simulink model "BESSmodel_EMT"  (R2019a)
settings: Solver=FixedStepAuto  SolverName=VariableStepAuto  StartTime=0.0  StopTime=10  RelTol=1e-3
undefined symbols (not defined in the file): D11, Delta, Ion, Lithium
libraries: powerlib x24, powerlib_meascontrol x15, simulink x9, eeGeneralControl x8, electricdrivelib x1
(part 1 of 2)
settings Model: Creator=rodne  LastModifiedBy=iq22022
settings DebuggingCC: UnderspecifiedInitializationDetection=Classic  MergeDetectMultiDrivingBlocksExec=none  UnconnectedInputMsg=none  UnconnectedOutputMsg=none  UnconnectedLineMsg=none  SFMachineParentedDataDiag=error
settings ModelReferenceCC: PropagateSignalLabelsOutOfModel=off

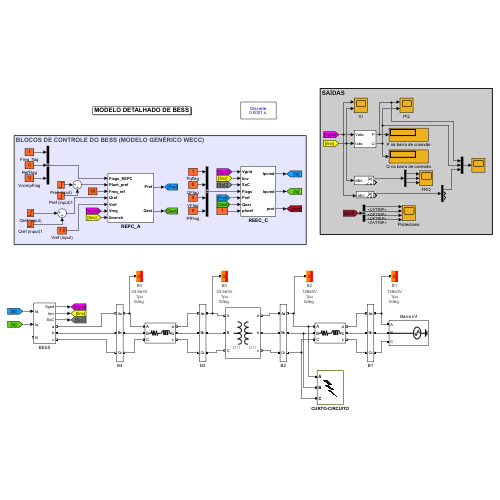
[thumbnail: Simulink's stored preview of the top-level diagram]
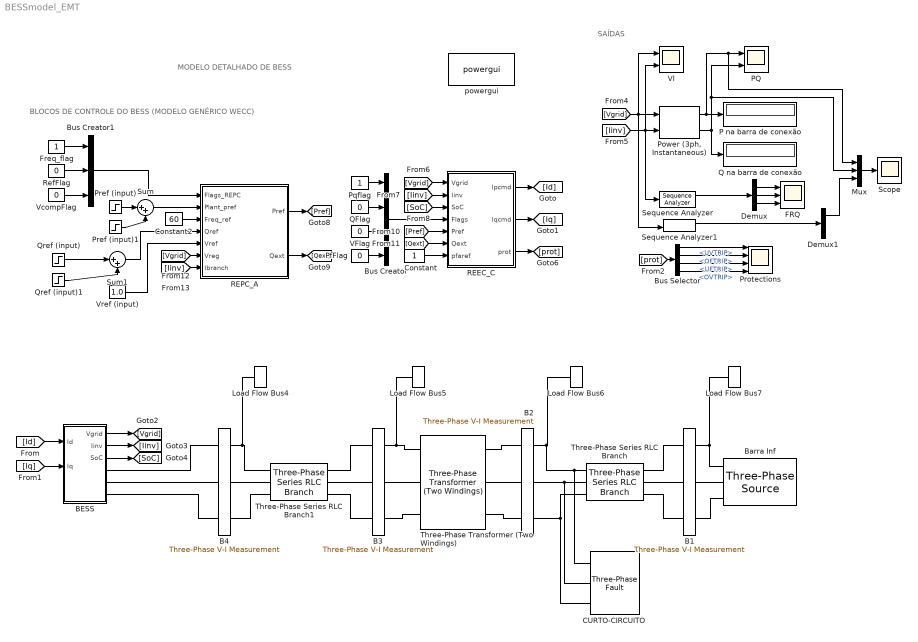
== system BESSmodel_EMT ==
  note: MODELO DETALHADO DE BESS
  note: SAÍDAS
  note: BLOCOS DE CONTROLE DO BESS (MODELO GENÉRICO WECC)
  B{1..4} (4 alike) : powerlib/Measurements/Three-Phase V-I Measurement  VoltageMeasurement=no  SetLabelV=off  LabelV=Vabc  Vpu=off  VpuLL=off  CurrentMeasurement=no  SetLabelI=off  LabelI=Iabc  Ipu=off  Pbase=100e6  Vbase=500e3  OutputType=Complex  PhasorSimulation=off  PSBequivalent=0
  BESS : Subsystem
  Barra Inf : powerlib/Electrical Sources/Three-Phase Source  InternalConnection=Yg  VoltagePhases=off  Voltage=138e3  PhaseAngle=0  Voltage_phases=[25e3 25e3 25e3]/sqrt(3)  PhaseAngles_phases=[0 -120 +120]  Frequency=60  NonIdealSource=off  SpecifyImpedance=off  Resistance=0.8929  Inductance=16.58e-3  ShortCircuitLevel=100e6  BaseVoltage=138e3  XRratio=7  BusType=swing  Pref=10e3  Qref=0  Prefabc=[10e3, 10e3, 10e3]  Qrefabc=[0, 0, 0]  Qmin=-inf  Qmax=inf
  Bus Creator : BusCreator  Inputs=4
  Bus Creator1 : BusCreator  Inputs=3
  Bus Selector : BusSelector  OutputSignals=UVTRIP,OFTRIP,UFTRIP,OVTRIP
  CURTO-CIRCUITO : powerlib/Elements/Three-Phase Fault  InitialStates=0  FaultA=on  FaultB=off  FaultC=off  GroundFault=on  SwitchTimes="[5.0  6.0]"  External=off  SwitchStatus=NaN  FaultResistance=60  GroundResistance=0.01  SnubberResistance=1e6  SnubberCapacitance=inf  Measurements=None
  Constant : Constant
  Constant2 : Constant  Value=60
  Demux : Demux  Outputs=3
  Demux1 : Demux  Outputs=3
  FRQ : Scope  NumInputPorts=3
  Freq_flag : Constant
  Load Flow Bus4 : powerlib/Measurements/Load Flow Bus  LConnTagsString=a  Phases=single  Connectors=on one side  ID=B4  Vbase=34.5e3  Vref=0.97  Vangle=0  VLF=1  VLFb=1  VLFc=1  angleLF=0  angleLFb=0  angleLFc=0
  Load Flow Bus5 : powerlib/Measurements/Load Flow Bus  LConnTagsString=a  Phases=single  Connectors=on one side  ID=B3  Vbase=34.5e3  Vref=1  Vangle=0  VLF=1  VLFb=1  VLFc=1  angleLF=0  angleLFb=0  angleLFc=0
  Load Flow Bus6 : powerlib/Measurements/Load Flow Bus  LConnTagsString=a  Phases=single  Connectors=on one side  ID=B2  Vbase=138e3  Vref=1  Vangle=0  VLF=1  VLFb=1  VLFc=1  angleLF=0  angleLFb=0  angleLFc=0
  Load Flow Bus7 : powerlib/Measurements/Load Flow Bus  LConnTagsString=a  Phases=single  Connectors=on one side  ID=B1  Vbase=138e3  Vref=1  Vangle=0  VLF=1  VLFb=1  VLFc=1  angleLF=0  angleLFb=0  angleLFc=0
  Mux : Mux  Inputs=3
  P na barra de conexão : Display
  PQ : Scope  NumInputPorts=2
  PfFlag : Constant  Value=0
  "Power (3ph, Instantaneous)" : powerlib_meascontrol/Measurements/Power (3ph, Instantaneous)
  Pqflag : Constant
  Pref (input) : Step  After=1.0  SampleTime=0
  Pref (input)1 : Step  Time=10  After=0  SampleTime=0
  Protections : Scope  NumInputPorts=4
  Q na barra de conexão : Display
  QFlag : Constant  Value=0
  Qref (input) : Step  Time=15  After=0  SampleTime=0
  Qref (input)1 : Step  Time=25  After=0  SampleTime=0
  REEC_C : Subsystem
  REPC_A : Subsystem
  RefFlag : Constant  Value=0
  Scope : Scope
  Sequence Analyzer : powerlib_meascontrol/Measurements/Sequence Analyzer  Freq=60  n=1  seq=Positive Negative Zero  InInit=[1, 0]  Ts=0
      settings: SourceProductBaseCode=PS
  Sequence Analyzer1 : powerlib_meascontrol/Measurements/Sequence Analyzer  Freq=60  n=1  seq=Positive Negative Zero  InInit=[1, 0]  Ts=0
      settings: SourceProductBaseCode=PS
  Sum : Sum  Inputs=|++
  Sum1 : Sum  Inputs=|++
  Three-Phase Series RLC Branch : powerlib/Elements/Three-Phase Series RLC Branch  LConnTagsString=A|B|C  RConnTagsString=A|B|C  BranchType=RL  Resistance=28.1667  Inductance=281.6667/(2*pi*60)  Capacitance=1e-6  Measurements=None
  Three-Phase Series RLC Branch1 : powerlib/Elements/Three-Phase Series RLC Branch  LConnTagsString=A|B|C  RConnTagsString=A|B|C  BranchType=RL  Resistance=0.0119  Inductance=0.1190/(2*pi*60)  Capacitance=1e-6  Measurements=None
  Three-Phase Transformer (Two Windings) : powerlib/Elements/Three-Phase Transformer (Two Windings)  Winding1Connection=Delta (D11)  Winding2Connection=Delta (D11)  CoreType=Three single-phase transformers  SetSaturation=off  Hysteresis=off  DataFile='hysteresis'  SetInitialFlux=off  Measurements=None  UNITS=pu  NominalPower=[ 6e6 , 60 ]  Winding1=[34.5e+03 0.0001/2 0.06/(2*pi*60)/2]  Winding2=[138e+03 0.0001/2 0.06/(2*pi*60)/2]  Rm=499.98  Lm=500  L0=0.5  Saturation=[0 0;0.0024 1.2;1 1.52]  InitialFluxes=[ 0.8 , -0.8 , 0.7 ]  BreakLoop=off  DiscreteSolver=Trapezoidal iterative  DataType=off  TransfoNumber=1
  VFlag : Constant  Value=0
  VI : Scope  NumInputPorts=2
  VcompFlag : Constant  Value=0
  Vref (input) : Constant  Value=1.0
  powergui : powerlib/powergui  Priority=1  SimulationMode=Discrete  SampleTime=100e-6  frequency=60  Iterations=50  frequencyindice=60  Pbase=100e6  ErrMax=1e-4  UnitsV=kV  UnitsW=MW  buscounter=0  FunctionMessages=off  echomessages=off  EnableUseOfTLC=off  CurrentSourceSwitches=off  DisableSnubberDevices=off  DisableRonSwitches=off  DisableVfSwitches=off  DisplayEquations=off  AutomaticDiscreteSolvers=off  SolverType=Tustin/Backward Euler (TBE)  Interpol=off  ExternalGateDelay=off  methode=off  Ts=100  x0status=blocks  SPID=on  SwTol=0  HookPort=off  NonlinearTolerance=1e-4  nMaxIteration=100  ContinueOnMaxIteration=off  RestoreLinks=warning  ResistiveCurrentMeasurement=off  Frange=[0:2:500]  Ylog=off  Xlog=on  ShowGrid=off  save=off  variable=ZData  structure=0  ZoomFFT=off  StartTime=0.0  cycles=1  DisplayStyle=1  fundamental=60  FreqAxis=off  MaxFrequency=1000  frequencyindicesteady=1  RmsSteady=1  display=off
  wires:
  "Power (3ph, Instantaneous)"/1 -> Mux/1, PQ/1, P na barra de conexão/1
  "Power (3ph, Instantaneous)"/2 -> PQ/2, Mux/2, Q na barra de conexão/1
  REEC_C/1(Ipcmd) -> [Id]
  REEC_C/2(Iqcmd) -> [Iq]
  [Vgrid] -> Sequence Analyzer1/1, VI/1, "Power (3ph, Instantaneous)"/1
  [Iinv] -> Sequence Analyzer/1, VI/2, "Power (3ph, Instantaneous)"/2
  [Vgrid] -> REEC_C/1(Vgrid)
  [Iinv] -> REEC_C/2(Iinv)
  [SoC] -> REEC_C/3(SoC)
  Pqflag/1 -> Bus Creator/1
  QFlag/1 -> Bus Creator/2
  PfFlag/1 -> Bus Creator/4
  VFlag/1 -> Bus Creator/3
  Bus Creator/1 -> REEC_C/4(Flags)
  Constant/1 -> REEC_C/7(pfaref)
  [Id] -> BESS/1(Id)
  [Iq] -> BESS/2(Iq)
  BESS/1(Vgrid) -> [Vgrid]
  BESS/2(Iinv) -> [Iinv]
  BESS/3(SoC) -> [SoC]
  Freq_flag/1 -> Bus Creator1/1
  RefFlag/1 -> Bus Creator1/2
  VcompFlag/1 -> Bus Creator1/3
  Bus Creator1/1 -> REPC_A/1(Flags_REPC)
  REPC_A/1(Pref) -> [Pref]
  REPC_A/2(Qext) -> [Qext]
  Constant2/1 -> REPC_A/3(Freq_ref)
  Vref (input)/1 -> REPC_A/5(Vref)
  [Pref] -> REEC_C/5(Pref)
  [Vgrid] -> REPC_A/6(Vreg)
  [Iinv] -> REPC_A/7(Ibranch)
  [Qext] -> REEC_C/6(Qext)
  REEC_C/3(prot) -> [prot]
  [prot] -> Bus Selector/1
  Bus Selector/1 -> Protections/1  "<UVTRIP>"
  Bus Selector/2 -> Protections/2  "<OFTRIP>"
  Bus Selector/3 -> Protections/3  "<UFTRIP>"
  Bus Selector/4 -> Protections/4  "<OVTRIP>"
  Sequence Analyzer/1 -> Demux/1
  Demux/1 -> FRQ/1
  Demux/2 -> FRQ/2
  Demux/3 -> FRQ/3
  Sum/1 -> REPC_A/2(Plant_pref)
  Pref (input)/1 -> Sum/1
  Pref (input)1/1 -> Sum/2
  Sum1/1 -> REPC_A/4(Qref)
  Qref (input)/1 -> Sum1/1
  Qref (input)1/1 -> Sum1/2
  Sequence Analyzer1/1 -> Demux1/1
  Mux/1 -> Scope/1
  Demux1/1 -> Mux/3
  connections:
  BESS/RConn1 -- B4/LConn1
  B4/LConn2 -- BESS/RConn2
  BESS/RConn3 -- B4/LConn3
  B3/RConn1 -- Load Flow Bus5/LConn1 -- Three-Phase Transformer (Two Windings)/LConn1
  Load Flow Bus7/LConn1 -- Barra Inf/RConn1 -- B1/RConn1
  B2/RConn1 -- CURTO-CIRCUITO/LConn1 -- Three-Phase Series RLC Branch/LConn1 -- Load Flow Bus6/LConn1
  B4/RConn1 -- Three-Phase Series RLC Branch1/LConn1 -- Load Flow Bus4/LConn1
  Three-Phase Series RLC Branch1/LConn2 -- B4/RConn2
  B3/RConn3 -- Three-Phase Transformer (Two Windings)/LConn3
  B3/RConn2 -- Three-Phase Transformer (Two Windings)/LConn2
  Three-Phase Series RLC Branch/RConn2 -- B1/LConn2
  Three-Phase Series RLC Branch1/RConn3 -- B3/LConn3
  B2/LConn3 -- Three-Phase Transformer (Two Windings)/RConn3
  B2/LConn1 -- Three-Phase Transformer (Two Windings)/RConn1
  Three-Phase Series RLC Branch/LConn2 -- CURTO-CIRCUITO/LConn2 -- B2/RConn2
  Three-Phase Series RLC Branch/RConn3 -- B1/LConn3
  Three-Phase Series RLC Branch1/RConn2 -- B3/LConn2
  Three-Phase Series RLC Branch1/RConn1 -- B3/LConn1
  Three-Phase Series RLC Branch/RConn1 -- B1/LConn1
  B2/LConn2 -- Three-Phase Transformer (Two Windings)/RConn2
  Three-Phase Series RLC Branch/LConn3 -- CURTO-CIRCUITO/LConn3 -- B2/RConn3
  Three-Phase Series RLC Branch1/LConn3 -- B4/RConn3
  Barra Inf/RConn2 -- B1/RConn2
  Barra Inf/RConn3 -- B1/RConn3

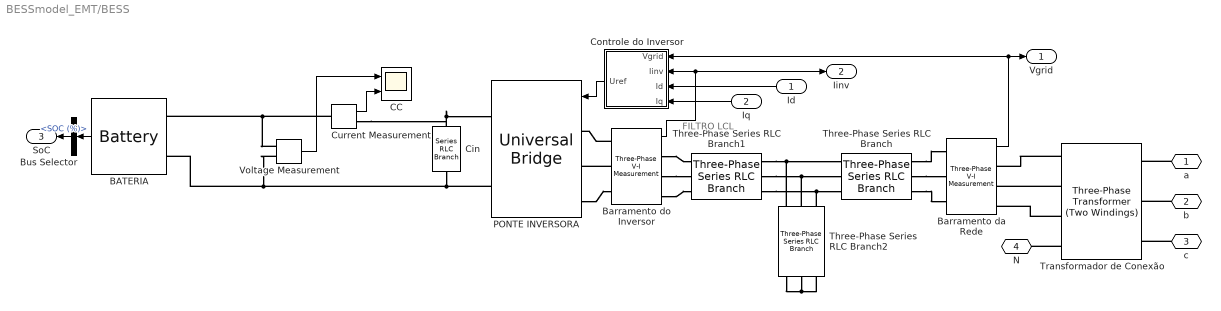
== system BESSmodel_EMT/BESS ==
  note: FILTRO LCL
  Id : Inport
  Iq : Inport  Port=2
  BATERIA : electricdrivelib/Extra Sources/Battery  BatType=Lithium-Ion  ShowTempParam=off  ThermalPreset=no  ShowAgeParam=off  NomV=1332  NomQ=280  SOC=70  Batt_Tr=30  PresetModel=off  MaxQ=280  MinV=999  FullV=1550.4309  Dis_rate=121.7391  R=0.047571*2.0  Normal_OP=253.2174  expZone="[1439.074      13.756522]"  current=[6.5 13 32.5]  Units=Time  Tci=20  NomT=20  T2=-30  MaxQ2=4.8  FullV2=7.1  Normal_OP2=5.655  expZone2="[6.58           1]"  Rca=0.6  ti=2000  Dp=0  Neq0=0  Tsim=1e6  Ta1=25  Qeol=5.4*0.9  Reol=0.013333*1.2  Char_age=[2.3478, 3]  Dis_age=[2.3478, 10]  N1=1500  N2=10500  N3=1000  N4=1400  Ta2=45  N5=950
  Barramento da Rede : powerlib/Measurements/Three-Phase V-I Measurement  VoltageMeasurement=phase-to-phase  SetLabelV=off  LabelV=Vabc  Vpu=off  VpuLL=on  CurrentMeasurement=no  SetLabelI=off  LabelI=Iabc  Ipu=off  Pbase=100e6  Vbase=690  OutputType=Complex  PhasorSimulation=off  PSBequivalent=0
  Barramento do Inversor : powerlib/Measurements/Three-Phase V-I Measurement  VoltageMeasurement=no  SetLabelV=off  LabelV=Vabc  Vpu=off  VpuLL=off  CurrentMeasurement=yes  SetLabelI=off  LabelI=Iabc  Ipu=on  Pbase=100e6  Vbase=690e3  OutputType=Complex  PhasorSimulation=off  PSBequivalent=0
  Bus Selector : BusSelector  OutputSignals=SOC (%)
  CC : Scope  NumInputPorts=2
  Cin : powerlib/Elements/Series RLC Branch  LConnTagsString=__new0  RConnTagsString=__new0  BranchType=RC  Resistance=0.0025  Inductance=1e-3  SetiL0=off  InitialCurrent=0  Capacitance=100e-6  Setx0=off  InitialVoltage=0  Measurements=None
  Controle do Inversor : Subsystem  mask(Direct-Quadrature Synchronous Reference Frame Controller){VDC=1332, f=60, fsw=10000, L=1000e-6, kp=5, ki=5000}
      mask prompts: VDC "DC Link Voltage (V)"; f "Grid Frequency (Hz)"; fsw "Switching Frequency (Hz)"; L "Filter Inductance (H)"; kp "Proportional Gain"; ki "Integral Gain"
      mask help:
      | Developed by Rodney Tan (PhD)
      | Version 1.0 (Nov 2021)
      |
      | This model demonstrate the operation of 3 phase grid connected inverter using Direct-Quadrature Synchronous Reference Frame Control.
      |
      | SPWM is use to switch the IGBT inverter bridge.
      |
      | The controller allows user to set the DC link voltage, active and reactive current for the inverter to be injected to the grid.
      |
      | The scope monitor the grid inverter output voltage and current waveform.
      |
      | The display monitor the active and reactive power injected to the grid.
      mask DialogControl Container3 Prompt: PI Controller Setting
  Current Measurement : powerlib/Measurements/Current Measurement  PhasorSimulation=off  OutputType=Complex  PSBequivalent=0
  PONTE INVERSORA : powerlib/Power Electronics/Universal Bridge  Arms=3  SnubberResistance=1e5  SnubberCapacitance=inf  Device=Average-model based VSC  Ron=1e-3  Lon=0  ForwardVoltages="[  0  0  ]"  ForwardVoltage=0  GTOparameters=[ 10e-6 , 20e-6 ]  IGBTparameters=[ 1e-6 , 2e-6 ]  Measurements=None  Measurements_2=None  converterType=Rectifier
  Three-Phase Series RLC Branch : powerlib/Elements/Three-Phase Series RLC Branch  LConnTagsString=A|B|C  RConnTagsString=A|B|C  BranchType=L  Resistance=1  Inductance=500e-6  Capacitance=1e-6  Measurements=None
  Three-Phase Series RLC Branch1 : powerlib/Elements/Three-Phase Series RLC Branch  LConnTagsString=A|B|C  RConnTagsString=A|B|C  BranchType=L  Resistance=1  Inductance=500e-6  Capacitance=1e-6  Measurements=None
  Three-Phase Series RLC Branch2 : powerlib/Elements/Three-Phase Series RLC Branch  LConnTagsString=A|B|C  RConnTagsString=A|B|C  BranchType=C  Resistance=1  Inductance=1e-3  Capacitance=700e-6  Measurements=None
  Transformador de Conexão : powerlib/Elements/Three-Phase Transformer (Two Windings)  Winding1Connection=Yn  Winding2Connection=Delta (D11)  CoreType=Three single-phase transformers  SetSaturation=off  Hysteresis=off  DataFile='hysteresis'  SetInitialFlux=off  Measurements=None  UNITS=pu  NominalPower=[ 34.5e6 , 60 ]  Winding1=[ 690 , 0.002 , 0.08 ]  Winding2=[ 34.5e3 , 0.002 , 0.08 ]  Rm=500  Lm=500  L0=0.5  Saturation=[ 0,0 ; 0.0024,1.2 ; 1.0,1.52 ]  InitialFluxes=[ 0.8 , -0.8 , 0.7 ]  BreakLoop=off  DiscreteSolver=Trapezoidal iterative  DataType=off  TransfoNumber=1
  Voltage Measurement : powerlib/Measurements/Voltage Measurement  PhasorSimulation=off  OutputType=Complex  PSBequivalent=0
  a : PMIOPort  Side=Right
  b : PMIOPort  Port=2  Side=Right
  c : PMIOPort  Port=3  Side=Right
  N : PMIOPort  Port=4  Side=Left
  Vgrid : Outport
  Iinv : Outport  Port=2
  SoC : Outport  Port=3
  wires:
  Id/1 -> Controle do Inversor/3(Id)
  Bus Selector/1 -> SoC/1  "<SOC (%)>"
  Iq/1 -> Controle do Inversor/4(Iq)
  Barramento da Rede/1 -> Vgrid/1, Controle do Inversor/1(Vgrid)
  Controle do Inversor/1(Uref) -> PONTE INVERSORA/1
  BATERIA/1 -> Bus Selector/1
  Barramento do Inversor/1 -> Controle do Inversor/2(Iinv), Iinv/1
  Voltage Measurement/1 -> CC/1
  Current Measurement/1 -> CC/2
  connections:
  Three-Phase Series RLC Branch1/RConn3 -- Three-Phase Series RLC Branch/LConn3 -- Three-Phase Series RLC Branch2/LConn3
  Transformador de Conexão/LConn2 -- Barramento da Rede/RConn2
  Three-Phase Series RLC Branch1/RConn2 -- Three-Phase Series RLC Branch/LConn2 -- Three-Phase Series RLC Branch2/LConn2
  PONTE INVERSORA/LConn3 -- Barramento do Inversor/LConn3
  b/RConn1 -- Transformador de Conexão/RConn2
  PONTE INVERSORA/RConn2 -- Voltage Measurement/LConn2 -- BATERIA/LConn2 -- Cin/RConn1
  Three-Phase Series RLC Branch2/RConn1 -- Three-Phase Series RLC Branch2/RConn2 -- Three-Phase Series RLC Branch2/RConn3
  Transformador de Conexão/LConn1 -- Barramento da Rede/RConn1
  Cin/LConn1 -- Current Measurement/RConn1 -- PONTE INVERSORA/RConn1
  Three-Phase Series RLC Branch1/RConn1 -- Three-Phase Series RLC Branch/LConn1 -- Three-Phase Series RLC Branch2/LConn1
  Transformador de Conexão/LConn4 -- N/RConn1
  c/RConn1 -- Transformador de Conexão/RConn3
  Barramento do Inversor/LConn2 -- PONTE INVERSORA/LConn2
  Barramento do Inversor/RConn1 -- Three-Phase Series RLC Branch1/LConn1
  Barramento do Inversor/RConn3 -- Three-Phase Series RLC Branch1/LConn3
  Barramento do Inversor/RConn2 -- Three-Phase Series RLC Branch1/LConn2
  Three-Phase Series RLC Branch/RConn2 -- Barramento da Rede/LConn2
  a/RConn1 -- Transformador de Conexão/RConn1
  Barramento do Inversor/LConn1 -- PONTE INVERSORA/LConn1
  Three-Phase Series RLC Branch/RConn1 -- Barramento da Rede/LConn1
  Transformador de Conexão/LConn3 -- Barramento da Rede/RConn3
  Three-Phase Series RLC Branch/RConn3 -- Barramento da Rede/LConn3
  Current Measurement/LConn1 -- Voltage Measurement/LConn1 -- BATERIA/LConn1

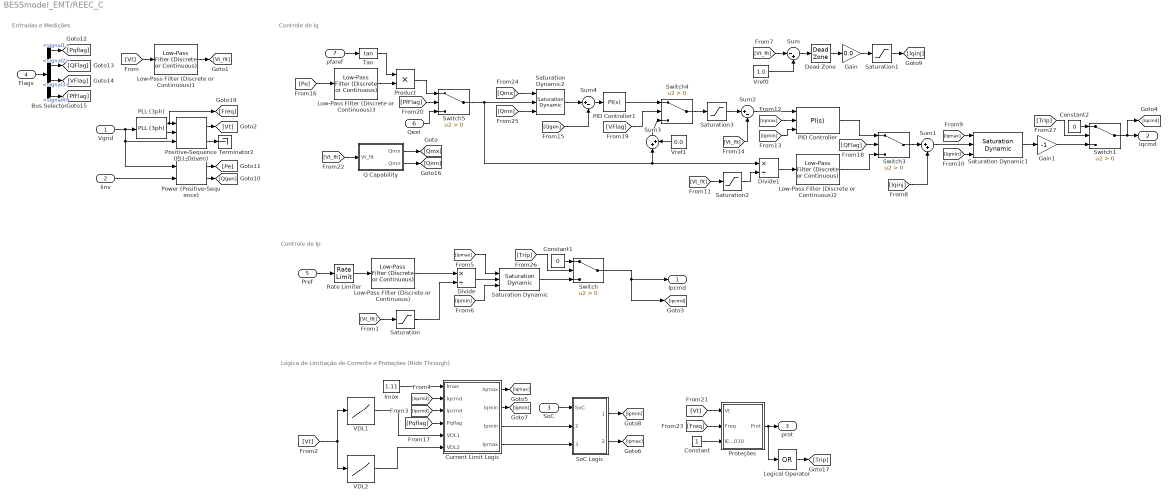
== system BESSmodel_EMT/REEC_C ==
  note: Entradas e Medições
  note: Controle de Iq
  note: Lógica de Limitação de Corrente e Proteções (Ride Through)
  note: Controle de Ip
  Vgrid : Inport
  Iinv : Inport  Port=2
  SoC : Inport  Port=3
  Flags : Inport  Port=4
  Pref : Inport  Port=5
  Qext : Inport  Port=6
  pfaref : Inport  Port=7
  Bus Selector : BusSelector  OutputSignals=signal1,signal2,signal3,signal4
  Constant : Constant
  Constant1 : Constant  Value=0
  Constant2 : Constant  Value=0
  Current Limit Logic : Subsystem
  Dead Zone : DeadZone  LowerValue=-0.05  UpperValue=0.05  SaturateOnIntegerOverflow=on
  Divide : Product  Inputs=*/
  Divide1 : Product  Inputs=*/
  Gain : Gain  Gain=0.0
  Gain1 : Gain  Gain=-1
  Imax : Constant  Value=1.11
  Logical Operator : Logic  Operator=OR  Inputs=1  AllPortsSameDT=off  OutDataTypeStr=boolean
  Low-Pass Filter (Discrete or Continuous) : eeGeneralControl/Low-Pass Filter (Discrete or Continuous)  K=1  T=0.017  B=inf  A=-inf  init_option=Inherited from block input  x0=0  Ts=0
  Low-Pass Filter (Discrete or Continuous)1 : eeGeneralControl/Low-Pass Filter (Discrete or Continuous)  K=1  T=0.01  B=inf  A=-inf  init_option=Inherited from block input  x0=0  Ts=0
  Low-Pass Filter (Discrete or Continuous)2 : eeGeneralControl/Low-Pass Filter (Discrete or Continuous)  K=1  T=0.017  B=inf  A=-inf  init_option=Inherited from block input  x0=0  Ts=0
  Low-Pass Filter (Discrete or Continuous)3 : eeGeneralControl/Low-Pass Filter (Discrete or Continuous)  K=1  T=0.05  B=inf  A=-inf  init_option=Inherited from block input  x0=0  Ts=0
  PID Controller : simulink/Continuous/PID Controller  Controller=PI  Form=Parallel  TimeDomain=Continuous-time  SampleTime=-1  IntegratorMethod=Forward Euler  ControllerParametersSource=internal  P=1.0  I=1.0  D=0  N=100  UseFilter=on  TunerSelectOption=Transfer Function Based (PID Tuner App)  InitialConditionSource=internal  InitialConditionForIntegrator=0  InitialConditionForFilter=0  DifferentiatorICPrevScaledInput=0  ExternalReset=none  TrackingMode=off  Kt=1  LimitOutput=on  UpperSaturationLimit=inf  LowerSaturationLimit=-inf  LinearizeAsGain=on  AntiWindupMode=none  Kb=1  POutMin=[]  POutMax=[]  IOutMin=[]  IOutMax=[]  DOutMin=[]  DOutMax=[]  NOutMin=[]  NOutMax=[]  SumOutMin=[]  SumOutMax=[]  SaturationOutMin=[]  SaturationOutMax=[]  PParamMin=[]  PParamMax=[]  IParamMin=[]  IParamMax=[]  DParamMin=[]  DParamMax=[]  NParamMin=[]  NParamMax=[]  KbParamMin=[]  KbParamMax=[]  KtParamMin=[]  KtParamMax=[]  KbOutMin=[]  KbOutMax=[]  KtOutMin=[]  KtOutMax=[]  IntegratorOutMin=[]  IntegratorOutMax=[]  FilterOutMin=[]  FilterOutMax=[]  SumI1OutMin=[]  SumI1OutMax=[]  SumI2OutMin=[]  SumI2OutMax=[]  SumI3OutMin=[]  SumI3OutMax=[]  SumI4OutMin=[]  SumI4OutMax=[]  SumDOutMin=[]  SumDOutMax=[]  DifferentiatorOutMin=[]  DifferentiatorOutMax=[]  FilterDiffOutCoefMin=[]  FilterDiffOutCoefMax=[]  ReciprocalOutMin=[]  ReciprocalOutMax=[]  SumDenOutMin=[]  SumDenOutMax=[]  SumNumOutMin=[]  SumNumOutMax=[]  DivideOutMin=[]  DivideOutMax=[]  IntegratorContinuousStateAttributes=''  IntegratorStateMustResolveToSignalObject=off  IntegratorRTWStateStorageClass=Auto  FilterContinuousStateAttributes=''  FilterStateMustResolveToSignalObject=off  FilterRTWStateStorageClass=Auto  ParallelPVariant=InternalParameters  IdealPVariant=Disabled  IVariant=InternalParameters  DVariant=Disabled  IntegratorVariant=Continuous  SatVariant=External  AWVariant=Passthrough  PCopyVariant=Disabled  TRVariant=Disabled  FdbkBlocksVariant=Forward  IdealPFdbkVariant=Disabled  SatFdbkVariant=Disabled  DerivativeFilterVariant=Disabled  NVariant=Disabled  NCopyVariant=Disabled_SignalSpec  FilterICVariant=Disabled  IntegratorICVariant=InternalICs  ExternalResetVariant=Disabled  TRSumVariant=Passthrough  SumFdbkVariant=Disabled  SumVariant=Sum_PI
  PID Controller1 : simulink/Continuous/PID Controller  Controller=PI  Form=Parallel  TimeDomain=Continuous-time  SampleTime=-1  IntegratorMethod=Forward Euler  ControllerParametersSource=internal  P=1.0  I=1.0  D=0  N=100  UseFilter=on  TunerSelectOption=Transfer Function Based (PID Tuner App)  InitialConditionSource=internal  InitialConditionForIntegrator=0  InitialConditionForFilter=0  DifferentiatorICPrevScaledInput=0  ExternalReset=none  TrackingMode=off  Kt=1  LimitOutput=on  UpperSaturationLimit=1.1  LowerSaturationLimit=0.9  LinearizeAsGain=on  AntiWindupMode=none  Kb=1  POutMin=[]  POutMax=[]  IOutMin=[]  IOutMax=[]  DOutMin=[]  DOutMax=[]  NOutMin=[]  NOutMax=[]  SumOutMin=[]  SumOutMax=[]  SaturationOutMin=[]  SaturationOutMax=[]  PParamMin=[]  PParamMax=[]  IParamMin=[]  IParamMax=[]  DParamMin=[]  DParamMax=[]  NParamMin=[]  NParamMax=[]  KbParamMin=[]  KbParamMax=[]  KtParamMin=[]  KtParamMax=[]  KbOutMin=[]  KbOutMax=[]  KtOutMin=[]  KtOutMax=[]  IntegratorOutMin=[]  IntegratorOutMax=[]  FilterOutMin=[]  FilterOutMax=[]  SumI1OutMin=[]  SumI1OutMax=[]  SumI2OutMin=[]  SumI2OutMax=[]  SumI3OutMin=[]  SumI3OutMax=[]  SumI4OutMin=[]  SumI4OutMax=[]  SumDOutMin=[]  SumDOutMax=[]  DifferentiatorOutMin=[]  DifferentiatorOutMax=[]  FilterDiffOutCoefMin=[]  FilterDiffOutCoefMax=[]  ReciprocalOutMin=[]  ReciprocalOutMax=[]  SumDenOutMin=[]  SumDenOutMax=[]  SumNumOutMin=[]  SumNumOutMax=[]  DivideOutMin=[]  DivideOutMax=[]  IntegratorContinuousStateAttributes=''  IntegratorStateMustResolveToSignalObject=off  IntegratorRTWStateStorageClass=Auto  FilterContinuousStateAttributes=''  FilterStateMustResolveToSignalObject=off  FilterRTWStateStorageClass=Auto  ParallelPVariant=InternalParameters  IdealPVariant=Disabled  IVariant=InternalParameters  DVariant=Disabled  IntegratorVariant=Continuous  SatVariant=Enabled  AWVariant=Passthrough  PCopyVariant=Disabled  TRVariant=Disabled  FdbkBlocksVariant=Forward  IdealPFdbkVariant=Disabled  SatFdbkVariant=Disabled  DerivativeFilterVariant=Disabled  NVariant=Disabled  NCopyVariant=Disabled_SignalSpec  FilterICVariant=Disabled  IntegratorICVariant=InternalICs  ExternalResetVariant=Disabled  TRSumVariant=Passthrough  SumFdbkVariant=Disabled  SumVariant=Sum_PI
  PLL (3ph) : powerlib_meascontrol/PLL/PLL (3ph)  Fmin=45  Par_Init=[0, 60]  ParK=[180, 3200, 1]  TcD=1e-4  MaxRateChangeFreq=12  FilterCutOffFreq=25  Ts=0  AGC=on
  Positive-Sequence (PLL-Driven) : powerlib_meascontrol/Measurements/Positive-Sequence (PLL-Driven)  Finit=60  Fmin=45  InInit=[1, 0]  Ts=0
      settings: SourceProductBaseCode=PS
  Power (Positive-Sequence) : powerlib_meascontrol/Measurements/Power (Positive-Sequence)  Freq=60  Vinit=[0, 0]  Iinit=[0, 0]  Ts=0
      settings: SourceProductBaseCode=PS
  Product : Product
  Proteções : Subsystem
  Q Capability : Subsystem
  Rate Limiter : RateLimiter  RisingSlewLimit=99  FallingSlewLimit=-99  SampleTimeMode=inherited
  Saturation : Saturate  UpperLimit=inf  LowerLimit=0.01
  Saturation Dynamic : simulink/Discontinuities/Saturation Dynamic  OutMin=[]  OutMax=[]  OutDataTypeStr=Inherit: Same as second input  OutDataType=fixdt(1, 16)  OutScaling=2^-10  DoSatur=off
  Saturation Dynamic1 : simulink/Discontinuities/Saturation Dynamic  OutMin=[]  OutMax=[]  OutDataTypeStr=Inherit: Same as second input  OutDataType=fixdt(1, 16)  OutScaling=2^-10  DoSatur=off
  Saturation Dynamic2 : simulink/Discontinuities/Saturation Dynamic  OutMin=[]  OutMax=[]  OutDataTypeStr=Inherit: Same as second input  OutDataType=fixdt(1, 16)  OutScaling=2^-10  DoSatur=off
  Saturation1 : Saturate  UpperLimit=0.75  LowerLimit=-0.75
  Saturation2 : Saturate  UpperLimit=inf  LowerLimit=0.01
  Saturation3 : Saturate  UpperLimit=1.1  LowerLimit=0.9
  SoC Logic : Subsystem
  Sum : Sum  Inputs=|-+
  Sum1 : Sum  Inputs=|++
  Sum2 : Sum  Inputs=|+-
  Sum3 : Sum  Inputs=|++
  Sum4 : Sum  Inputs=|+-
  Switch{,1,3..5} (5 alike) : Switch  Criteria=u2 > Threshold
  Tan : Trigonometry  Operator=tan
  Terminator2 : Terminator
  VDL1 : Lookup_n-D  NumberOfTableDimensions=1  BreakpointsForDimension1=[0;0.2;0.5;1]  Table=[0.75;0.750000001;0.750000002;0.750000003]  InternalRulePriority=Speed  RndMeth=Simplest  InputSameDT=on
  VDL2 : Lookup_n-D  NumberOfTableDimensions=1  BreakpointsForDimension1=[0.2;0.5;0.75;1]  Table=[1.11;1.110000001;1.110000002;1.110000003]  InternalRulePriority=Speed  RndMeth=Simplest  InputSameDT=on
  Vref0 : Constant  Value=1.0
  Vref1 : Constant  Value=0.0
  Ipcmd : Outport
  Iqcmd : Outport  Port=2
  prot : Outport  Port=3
  wires:
  Saturation Dynamic1/1 -> Gain1/1
  Pref/1 -> Rate Limiter/1
  Rate Limiter/1 -> Low-Pass Filter (Discrete or Continuous)/1
  Low-Pass Filter (Discrete or Continuous)/1 -> Divide/1
  [Vt] -> Low-Pass Filter (Discrete or Continuous)1/1
  Low-Pass Filter (Discrete or Continuous)1/1 -> [Vt_flt]
  [Vt_flt] -> Saturation/1
  Divide/1 -> Saturation Dynamic/2
  [Ipmax] -> Saturation Dynamic/1
  [Ipmin] -> Saturation Dynamic/3
  Vgrid/1 -> Power (Positive-Sequence)/1, Positive-Sequence (PLL-Driven)/3, PLL (3ph)/1
  Positive-Sequence (PLL-Driven)/1 -> [Vt]
  Positive-Sequence (PLL-Driven)/2 -> Terminator2/1
  PLL (3ph)/2 -> Positive-Sequence (PLL-Driven)/2
  PLL (3ph)/1 -> [Freq], Positive-Sequence (PLL-Driven)/1
  [Vt] -> VDL1/1, VDL2/1
  Imax/1 -> Current Limit Logic/1(Imax)
  [Iqcmd] -> Current Limit Logic/2(Iqcmd)
  [Ipcmd] -> Current Limit Logic/3(Ipcmd)
  [Pqflag] -> Current Limit Logic/4(Pqflag)
  VDL1/1 -> Current Limit Logic/5(VDL1)
  VDL2/1 -> Current Limit Logic/6(VDL2)
  Current Limit Logic/1(Iqmax) -> [Iqmax]
  Current Limit Logic/2(Iqmin) -> [Iqmin]
  Saturation/1 -> Divide/2
  [Vt_flt] -> Sum/1
  Vref0/1 -> Sum/2
  Sum/1 -> Dead Zone/1
  Dead Zone/1 -> Gain/1
  Gain/1 -> Saturation1/1
  Saturation1/1 -> [Iqinj]
  Low-Pass Filter (Discrete or Continuous)2/1 -> Switch3/3
  Switch3/1 -> Sum1/1
  [Iqinj] -> Sum1/2
  Sum1/1 -> Saturation Dynamic1/2
  [Iqmax] -> Saturation Dynamic1/1
  [Iqmin] -> Saturation Dynamic1/3
  Divide1/1 -> Low-Pass Filter (Discrete or Continuous)2/1
  [Vt_flt] -> Saturation2/1
  Saturation2/1 -> Divide1/2
  PID Controller/1 -> Switch3/1
  [Iqmax] -> PID Controller/2
  [Iqmin] -> PID Controller/3
  Sum2/1 -> PID Controller/1
  [Vt_flt] -> Sum2/2
  Saturation3/1 -> Sum2/1
  Switch4/1 -> Saturation3/1
  Sum3/1 -> Switch4/3
  Vref1/1 -> Sum3/2
  PID Controller1/1 -> Switch4/1
  Sum4/1 -> PID Controller1/1
  Iinv/1 -> Power (Positive-Sequence)/2
  Power (Positive-Sequence)/1 -> [Pe]
  Power (Positive-Sequence)/2 -> [Qgen]
  [Qgen] -> Sum4/2
  Switch5/1 -> Saturation Dynamic2/2, Divide1/1, Sum3/1
  Qext/1 -> Switch5/3
  [Pe] -> Low-Pass Filter (Discrete or Continuous)3/1
  Low-Pass Filter (Discrete or Continuous)3/1 -> Product/2
  Product/1 -> Switch5/1
  Tan/1 -> Product/1
  pfaref/1 -> Tan/1
  Flags/1 -> Bus Selector/1
  Bus Selector/1 -> [Pqflag]  "<signal1>"
  Bus Selector/2 -> [QFlag]  "<signal2>"
  Bus Selector/3 -> [VFlag]  "<signal3>"
  Bus Selector/4 -> [PfFlag]  "<signal4>"
  [QFlag] -> Switch3/2
  [VFlag] -> Switch4/2
  [PfFlag] -> Switch5/2
  [Vt] -> Proteções/1(Vt)
  [Freq] -> Proteções/2(Freq)
  Proteções/1(Prot) -> Logical Operator/1, prot/1
  Saturation Dynamic2/1 -> Sum4/1
  [Vt_flt] -> Q Capability/1(Vt_flt)
  Q Capability/1(Qmx) -> [Qmx]
  Q Capability/2(Qmn) -> [Qmn]
  [Qmx] -> Saturation Dynamic2/1
  [Qmn] -> Saturation Dynamic2/3
  SoC/1 -> SoC Logic/1(SoC)
  Current Limit Logic/3(Ipmin) -> SoC Logic/2(Ipmn)
  Current Limit Logic/4(Ipmax) -> SoC Logic/3(Ipmx)
  SoC Logic/1(Ipmin) -> [Ipmin]
  SoC Logic/2(Ipmax) -> [Ipmax]
  Constant/1 -> Proteções/3(IEEE2030)
  Logical Operator/1 -> [Trip]
  [Trip] -> Switch/2
  Switch/1 -> [Ipcmd], Ipcmd/1
  Saturation Dynamic/1 -> Switch/3
  Constant1/1 -> Switch/1
  Gain1/1 -> Switch1/3
  Constant2/1 -> Switch1/1
  [Trip] -> Switch1/2
  Switch1/1 -> [Iqcmd], Iqcmd/1

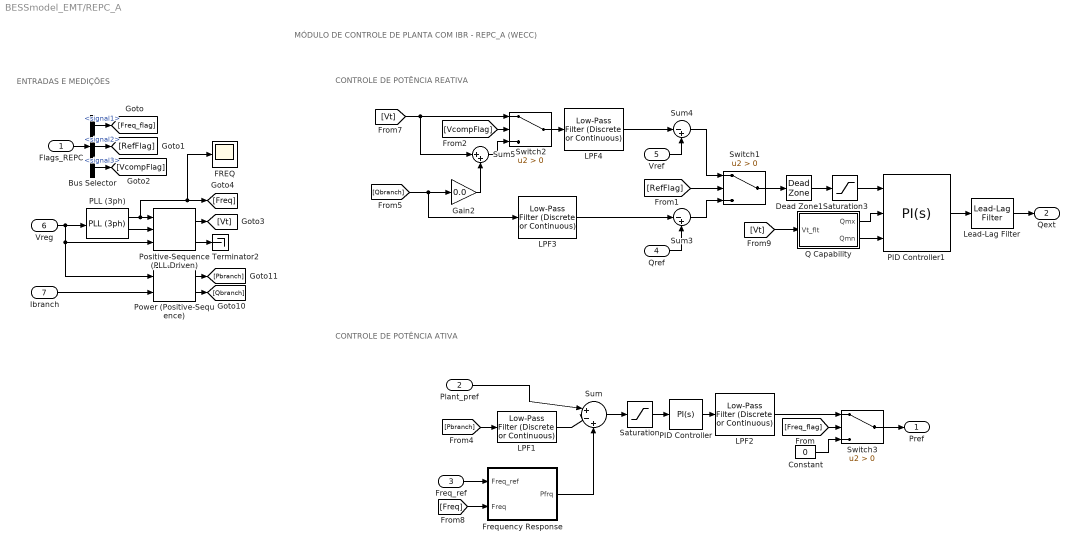
== system BESSmodel_EMT/REPC_A ==
  note: MÓDULO DE CONTROLE DE PLANTA COM IBR - REPC_A (WECC)
  note: ENTRADAS E MEDIÇÕES
  note: CONTROLE DE POTÊNCIA ATIVA
  note: CONTROLE DE POTÊNCIA REATIVA
  Flags_REPC : Inport
  Plant_pref : Inport  Port=2
  Freq_ref : Inport  Port=3
  Qref : Inport  Port=4
  Vref : Inport  Port=5
  Vreg : Inport  Port=6
  Ibranch : Inport  Port=7
  Bus Selector : BusSelector  OutputSignals=signal1,signal2,signal3
  Constant : Constant  Value=0
  Dead Zone1 : DeadZone  LowerValue=0.0  UpperValue=0.0  SaturateOnIntegerOverflow=on
  FREQ : Scope
  Frequency Response : Subsystem
  Gain2 : Gain  Gain=0.0
  LPF1 : eeGeneralControl/Low-Pass Filter (Discrete or Continuous)  K=1  T=0.25  B=inf  A=-inf  init_option=Inherited from block input  x0=0  Ts=0
  LPF2 : eeGeneralControl/Low-Pass Filter (Discrete or Continuous)  K=1  T=0.8  B=inf  A=-inf  init_option=Inherited from block input  x0=0  Ts=0
  LPF3 : eeGeneralControl/Low-Pass Filter (Discrete or Continuous)  K=1  T=0.02  B=inf  A=-inf  init_option=Inherited from block input  x0=0  Ts=0
  LPF4 : eeGeneralControl/Low-Pass Filter (Discrete or Continuous)  K=1  T=0.02  B=inf  A=-inf  init_option=Inherited from block input  x0=0  Ts=0
  Lead-Lag Filter : powerlib_meascontrol/Filters/Lead-Lag Filter  T1=0.01  T2=0.2  Vdc_Init=0  Ts=0
      settings: SourceProductBaseCode=PS
  PID Controller : simulink/Continuous/PID Controller  Controller=PI  Form=Parallel  TimeDomain=Continuous-time  SampleTime=-1  IntegratorMethod=Forward Euler  ControllerParametersSource=internal  P=1.0  I=1.0  D=0  N=100  UseFilter=on  TunerSelectOption=Transfer Function Based (PID Tuner App)  InitialConditionSource=internal  InitialConditionForIntegrator=0  InitialConditionForFilter=0  DifferentiatorICPrevScaledInput=0  ExternalReset=none  TrackingMode=off  Kt=1  LimitOutput=on  UpperSaturationLimit=1.0  LowerSaturationLimit=-0.667  LinearizeAsGain=on  AntiWindupMode=none  Kb=1  POutMin=[]  POutMax=[]  IOutMin=[]  IOutMax=[]  DOutMin=[]  DOutMax=[]  NOutMin=[]  NOutMax=[]  SumOutMin=[]  SumOutMax=[]  SaturationOutMin=[]  SaturationOutMax=[]  PParamMin=[]  PParamMax=[]  IParamMin=[]  IParamMax=[]  DParamMin=[]  DParamMax=[]  NParamMin=[]  NParamMax=[]  KbParamMin=[]  KbParamMax=[]  KtParamMin=[]  KtParamMax=[]  KbOutMin=[]  KbOutMax=[]  KtOutMin=[]  KtOutMax=[]  IntegratorOutMin=[]  IntegratorOutMax=[]  FilterOutMin=[]  FilterOutMax=[]  SumI1OutMin=[]  SumI1OutMax=[]  SumI2OutMin=[]  SumI2OutMax=[]  SumI3OutMin=[]  SumI3OutMax=[]  SumI4OutMin=[]  SumI4OutMax=[]  SumDOutMin=[]  SumDOutMax=[]  DifferentiatorOutMin=[]  DifferentiatorOutMax=[]  FilterDiffOutCoefMin=[]  FilterDiffOutCoefMax=[]  ReciprocalOutMin=[]  ReciprocalOutMax=[]  SumDenOutMin=[]  SumDenOutMax=[]  SumNumOutMin=[]  SumNumOutMax=[]  DivideOutMin=[]  DivideOutMax=[]  IntegratorContinuousStateAttributes=''  IntegratorStateMustResolveToSignalObject=off  IntegratorRTWStateStorageClass=Auto  FilterContinuousStateAttributes=''  FilterStateMustResolveToSignalObject=off  FilterRTWStateStorageClass=Auto  ParallelPVariant=InternalParameters  IdealPVariant=Disabled  IVariant=InternalParameters  DVariant=Disabled  IntegratorVariant=Continuous  SatVariant=Enabled  AWVariant=Passthrough  PCopyVariant=Disabled  TRVariant=Disabled  FdbkBlocksVariant=Forward  IdealPFdbkVariant=Disabled  SatFdbkVariant=Disabled  DerivativeFilterVariant=Disabled  NVariant=Disabled  NCopyVariant=Disabled_SignalSpec  FilterICVariant=Disabled  IntegratorICVariant=InternalICs  ExternalResetVariant=Disabled  TRSumVariant=Passthrough  SumFdbkVariant=Disabled  SumVariant=Sum_PI
  PID Controller1 : simulink/Continuous/PID Controller  Controller=PI  Form=Parallel  TimeDomain=Continuous-time  SampleTime=-1  IntegratorMethod=Forward Euler  ControllerParametersSource=internal  P=1.0  I=4.0  D=0  N=100  UseFilter=on  TunerSelectOption=Transfer Function Based (PID Tuner App)  InitialConditionSource=internal  InitialConditionForIntegrator=0  InitialConditionForFilter=0  DifferentiatorICPrevScaledInput=0  ExternalReset=none  TrackingMode=off  Kt=1  LimitOutput=on  UpperSaturationLimit=0.75  LowerSaturationLimit=-0.75  LinearizeAsGain=on  AntiWindupMode=none  Kb=1  POutMin=[]  POutMax=[]  IOutMin=[]  IOutMax=[]  DOutMin=[]  DOutMax=[]  NOutMin=[]  NOutMax=[]  SumOutMin=[]  SumOutMax=[]  SaturationOutMin=[]  SaturationOutMax=[]  PParamMin=[]  PParamMax=[]  IParamMin=[]  IParamMax=[]  DParamMin=[]  DParamMax=[]  NParamMin=[]  NParamMax=[]  KbParamMin=[]  KbParamMax=[]  KtParamMin=[]  KtParamMax=[]  KbOutMin=[]  KbOutMax=[]  KtOutMin=[]  KtOutMax=[]  IntegratorOutMin=[]  IntegratorOutMax=[]  FilterOutMin=[]  FilterOutMax=[]  SumI1OutMin=[]  SumI1OutMax=[]  SumI2OutMin=[]  SumI2OutMax=[]  SumI3OutMin=[]  SumI3OutMax=[]  SumI4OutMin=[]  SumI4OutMax=[]  SumDOutMin=[]  SumDOutMax=[]  DifferentiatorOutMin=[]  DifferentiatorOutMax=[]  FilterDiffOutCoefMin=[]  FilterDiffOutCoefMax=[]  ReciprocalOutMin=[]  ReciprocalOutMax=[]  SumDenOutMin=[]  SumDenOutMax=[]  SumNumOutMin=[]  SumNumOutMax=[]  DivideOutMin=[]  DivideOutMax=[]  IntegratorContinuousStateAttributes=''  IntegratorStateMustResolveToSignalObject=off  IntegratorRTWStateStorageClass=Auto  FilterContinuousStateAttributes=''  FilterStateMustResolveToSignalObject=off  FilterRTWStateStorageClass=Auto  ParallelPVariant=InternalParameters  IdealPVariant=Disabled  IVariant=InternalParameters  DVariant=Disabled  IntegratorVariant=Continuous  SatVariant=External  AWVariant=Passthrough  PCopyVariant=Disabled  TRVariant=Disabled  FdbkBlocksVariant=Forward  IdealPFdbkVariant=Disabled  SatFdbkVariant=Disabled  DerivativeFilterVariant=Disabled  NVariant=Disabled  NCopyVariant=Disabled_SignalSpec  FilterICVariant=Disabled  IntegratorICVariant=InternalICs  ExternalResetVariant=Disabled  TRSumVariant=Passthrough  SumFdbkVariant=Disabled  SumVariant=Sum_PI
  PLL (3ph) : powerlib_meascontrol/PLL/PLL (3ph)  Fmin=45  Par_Init=[0, 60]  ParK=[180, 3200, 1]  TcD=1e-4  MaxRateChangeFreq=12  FilterCutOffFreq=25  Ts=0  AGC=on
  Positive-Sequence (PLL-Driven) : powerlib_meascontrol/Measurements/Positive-Sequence (PLL-Driven)  Finit=60  Fmin=45  InInit=[1, 0]  Ts=0
      settings: SourceProductBaseCode=PS
  Power (Positive-Sequence) : powerlib_meascontrol/Measurements/Power (Positive-Sequence)  Freq=60  Vinit=[0, 0]  Iinit=[0, 0]  Ts=0
      settings: SourceProductBaseCode=PS
  Q Capability : Subsystem
  Saturation : Saturate  UpperLimit=99  LowerLimit=-99
  Saturation3 : Saturate  UpperLimit=1.0  LowerLimit=-1.0
  Sum : Sum  Inputs=|+-+
  Sum3 : Sum  Inputs=|-+
  Sum4 : Sum  Inputs=|-+
  Sum5 : Sum  Inputs=|++
  Switch1 : Switch  Criteria=u2 > Threshold
  Switch2 : Switch  Criteria=u2 > Threshold
  Switch3 : Switch  Criteria=u2 > Threshold
  Terminator2 : Terminator
  Pref : Outport
  Qext : Outport  Port=2
  wires:
  Switch3/1 -> Pref/1
  LPF2/1 -> Switch3/1
  PID Controller/1 -> LPF2/1
  Saturation/1 -> PID Controller/1
  Sum/1 -> Saturation/1
  Plant_pref/1 -> Sum/1
  [Pbranch] -> LPF1/1
  LPF1/1 -> Sum/2
  Lead-Lag Filter/1 -> Qext/1
  PID Controller1/1 -> Lead-Lag Filter/1
  Saturation3/1 -> PID Controller1/1
  Dead Zone1/1 -> Saturation3/1
  Switch1/1 -> Dead Zone1/1
  Flags_REPC/1 -> Bus Selector/1
  Bus Selector/1 -> [Freq_flag]  "<signal1>"
  Bus Selector/2 -> [RefFlag]  "<signal2>"
  Bus Selector/3 -> [VcompFlag]  "<signal3>"
  [Freq_flag] -> Switch3/2
  [RefFlag] -> Switch1/2
  Sum3/1 -> Switch1/3
  Qref/1 -> Sum3/2
  [Qbranch] -> LPF3/1, Gain2/1
  LPF3/1 -> Sum3/1
  Sum4/1 -> Switch1/1
  Vref/1 -> Sum4/2
  LPF4/1 -> Sum4/1
  Switch2/1 -> LPF4/1
  [VcompFlag] -> Switch2/2
  Sum5/1 -> Switch2/3
  Gain2/1 -> Sum5/2
  Constant/1 -> Switch3/3
  Power (Positive-Sequence)/2 -> [Qbranch]
  Power (Positive-Sequence)/1 -> [Pbranch]
  PLL (3ph)/1 -> FREQ/1, [Freq], Positive-Sequence (PLL-Driven)/1
  PLL (3ph)/2 -> Positive-Sequence (PLL-Driven)/2
  Positive-Sequence (PLL-Driven)/2 -> Terminator2/1
  Positive-Sequence (PLL-Driven)/1 -> [Vt]
  Vreg/1 -> PLL (3ph)/1, Positive-Sequence (PLL-Driven)/3, Power (Positive-Sequence)/1
  [Vt] -> Sum5/1, Switch2/1
  Ibranch/1 -> Power (Positive-Sequence)/2
  Freq_ref/1 -> Frequency Response/1(Freq_ref)
  [Freq] -> Frequency Response/2(Freq)
  Frequency Response/1(Pfrq) -> Sum/3
  Q Capability/1(Qmx) -> PID Controller1/2
  Q Capability/2(Qmn) -> PID Controller1/3
  [Vt] -> Q Capability/1(Vt_flt)

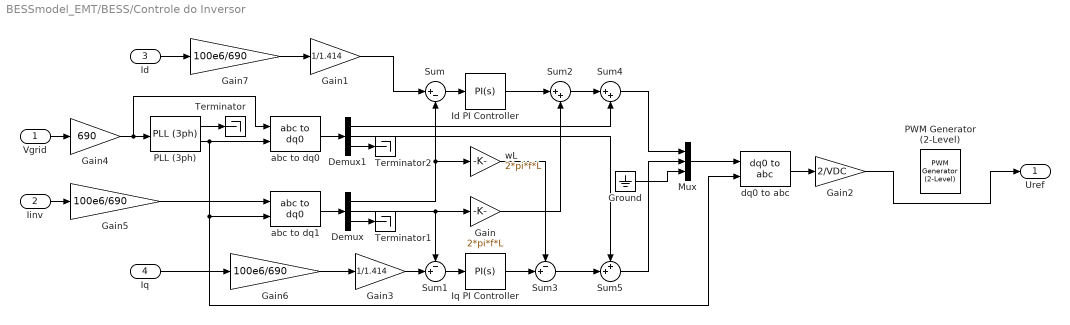
== system BESSmodel_EMT/BESS/Controle do Inversor ==
  Vgrid : Inport
  Iinv : Inport  Port=2
  Id : Inport  Port=3
  Iq : Inport  Port=4
  Demux : Demux  Outputs=3
  Demux1 : Demux  Outputs=3
  Gain : Gain  Gain=2*pi*f*L
  Gain1 : Gain  Gain=1/1.414
  Gain2 : Gain  Gain=2/VDC
  Gain3 : Gain  Gain=1/1.414
  Gain4 : Gain  Gain=690
  Gain5 : Gain  Gain=100e6/690
  Gain6 : Gain  Gain=100e6/690
  Gain7 : Gain  Gain=100e6/690
  Ground : Ground
  Id PI Controller : simulink/Continuous/PID Controller  Controller=PI  Form=Parallel  TimeDomain=Continuous-time  SampleTime=-1  IntegratorMethod=Forward Euler  ControllerParametersSource=internal  P=kp  I=ki  D=0  N=100  UseFilter=on  TunerSelectOption=Transfer Function Based (PID Tuner App)  InitialConditionSource=internal  InitialConditionForIntegrator=0  InitialConditionForFilter=0  DifferentiatorICPrevScaledInput=0  ExternalReset=none  TrackingMode=off  Kt=1  LimitOutput=off  UpperSaturationLimit=inf  LowerSaturationLimit=-inf  LinearizeAsGain=on  AntiWindupMode=none  Kb=1  POutMin=[]  POutMax=[]  IOutMin=[]  IOutMax=[]  DOutMin=[]  DOutMax=[]  NOutMin=[]  NOutMax=[]  SumOutMin=[]  SumOutMax=[]  SaturationOutMin=[]  SaturationOutMax=[]  PParamMin=[]  PParamMax=[]  IParamMin=[]  IParamMax=[]  DParamMin=[]  DParamMax=[]  NParamMin=[]  NParamMax=[]  KbParamMin=[]  KbParamMax=[]  KtParamMin=[]  KtParamMax=[]  KbOutMin=[]  KbOutMax=[]  KtOutMin=[]  KtOutMax=[]  IntegratorOutMin=[]  IntegratorOutMax=[]  FilterOutMin=[]  FilterOutMax=[]  SumI1OutMin=[]  SumI1OutMax=[]  SumI2OutMin=[]  SumI2OutMax=[]  SumI3OutMin=[]  SumI3OutMax=[]  SumI4OutMin=[]  SumI4OutMax=[]  SumDOutMin=[]  SumDOutMax=[]  DifferentiatorOutMin=[]  DifferentiatorOutMax=[]  FilterDiffOutCoefMin=[]  FilterDiffOutCoefMax=[]  ReciprocalOutMin=[]  ReciprocalOutMax=[]  SumDenOutMin=[]  SumDenOutMax=[]  SumNumOutMin=[]  SumNumOutMax=[]  DivideOutMin=[]  DivideOutMax=[]  IntegratorContinuousStateAttributes=''  IntegratorStateMustResolveToSignalObject=off  IntegratorRTWStateStorageClass=Auto  FilterContinuousStateAttributes=''  FilterStateMustResolveToSignalObject=off  FilterRTWStateStorageClass=Auto  ParallelPVariant=InternalParameters  IdealPVariant=Disabled  IVariant=InternalParameters  DVariant=Disabled  IntegratorVariant=Continuous  SatVariant=Disabled  AWVariant=Passthrough  PCopyVariant=Disabled  TRVariant=Disabled  FdbkBlocksVariant=Forward  IdealPFdbkVariant=Disabled  SatFdbkVariant=Disabled  DerivativeFilterVariant=Disabled  NVariant=Disabled  NCopyVariant=Disabled_SignalSpec  FilterICVariant=Disabled  IntegratorICVariant=InternalICs  ExternalResetVariant=Disabled  TRSumVariant=Passthrough  SumFdbkVariant=Disabled  SumVariant=Sum_PI
  Iq PI Controller : simulink/Continuous/PID Controller  Controller=PI  Form=Parallel  TimeDomain=Continuous-time  SampleTime=-1  IntegratorMethod=Forward Euler  ControllerParametersSource=internal  P=kp  I=ki  D=0  N=100  UseFilter=on  TunerSelectOption=Transfer Function Based (PID Tuner App)  InitialConditionSource=internal  InitialConditionForIntegrator=0  InitialConditionForFilter=0  DifferentiatorICPrevScaledInput=0  ExternalReset=none  TrackingMode=off  Kt=1  LimitOutput=off  UpperSaturationLimit=inf  LowerSaturationLimit=-inf  LinearizeAsGain=on  AntiWindupMode=none  Kb=1  POutMin=[]  POutMax=[]  IOutMin=[]  IOutMax=[]  DOutMin=[]  DOutMax=[]  NOutMin=[]  NOutMax=[]  SumOutMin=[]  SumOutMax=[]  SaturationOutMin=[]  SaturationOutMax=[]  PParamMin=[]  PParamMax=[]  IParamMin=[]  IParamMax=[]  DParamMin=[]  DParamMax=[]  NParamMin=[]  NParamMax=[]  KbParamMin=[]  KbParamMax=[]  KtParamMin=[]  KtParamMax=[]  KbOutMin=[]  KbOutMax=[]  KtOutMin=[]  KtOutMax=[]  IntegratorOutMin=[]  IntegratorOutMax=[]  FilterOutMin=[]  FilterOutMax=[]  SumI1OutMin=[]  SumI1OutMax=[]  SumI2OutMin=[]  SumI2OutMax=[]  SumI3OutMin=[]  SumI3OutMax=[]  SumI4OutMin=[]  SumI4OutMax=[]  SumDOutMin=[]  SumDOutMax=[]  DifferentiatorOutMin=[]  DifferentiatorOutMax=[]  FilterDiffOutCoefMin=[]  FilterDiffOutCoefMax=[]  ReciprocalOutMin=[]  ReciprocalOutMax=[]  SumDenOutMin=[]  SumDenOutMax=[]  SumNumOutMin=[]  SumNumOutMax=[]  DivideOutMin=[]  DivideOutMax=[]  IntegratorContinuousStateAttributes=''  IntegratorStateMustResolveToSignalObject=off  IntegratorRTWStateStorageClass=Auto  FilterContinuousStateAttributes=''  FilterStateMustResolveToSignalObject=off  FilterRTWStateStorageClass=Auto  ParallelPVariant=InternalParameters  IdealPVariant=Disabled  IVariant=InternalParameters  DVariant=Disabled  IntegratorVariant=Continuous  SatVariant=Disabled  AWVariant=Passthrough  PCopyVariant=Disabled  TRVariant=Disabled  FdbkBlocksVariant=Forward  IdealPFdbkVariant=Disabled  SatFdbkVariant=Disabled  DerivativeFilterVariant=Disabled  NVariant=Disabled  NCopyVariant=Disabled_SignalSpec  FilterICVariant=Disabled  IntegratorICVariant=InternalICs  ExternalResetVariant=Disabled  TRSumVariant=Passthrough  SumFdbkVariant=Disabled  SumVariant=Sum_PI
  Mux : Mux  Inputs=3
  PLL (3ph) : powerlib_meascontrol/PLL/PLL (3ph)  Fmin=45  Par_Init=[0, f]  ParK=[180, 3200, 1]  TcD=1e-4  MaxRateChangeFreq=12  FilterCutOffFreq=25  Ts=0  AGC=on
  PWM Generator (2-Level) : powerlib_meascontrol/Pulse & Signal Generators/PWM Generator (2-Level)  ModulatorType=Three-phase bridge (6 pulses)  ModulatorMode=Unsynchronized  Fc=fsw  Pc=0  nF=27  MinMax="[ -1  1 ]"  SamplingTechnique=Natural  ModulatingSignals=off  m=0.8  Freq=60  Phase=0  Ts=0  ShowCarrierOutport=off
  Sum : Sum  Inputs=|+-
  Sum1 : Sum  Inputs=-+|
  Sum2 : Sum  Inputs=|++
  Sum3 : Sum  Inputs=-+|
  Sum4 : Sum  Inputs=|++
  Sum5 : Sum  Inputs=++|
  Terminator : Terminator
  Terminator1 : Terminator
  Terminator2 : Terminator
  abc to dq0 : powerlib_meascontrol/Transformations/abc to dq0  Alignment=90 degrees behind phase A axis
  abc to dq1 : powerlib_meascontrol/Transformations/abc to dq0  Alignment=90 degrees behind phase A axis
  dq0 to abc : powerlib_meascontrol/Transformations/dq0 to abc  Alignment=90 degrees behind phase A axis
  wL : Gain  Gain=2*pi*f*L
  Uref : Outport
  wires:
  Id PI Controller/1 -> Sum2/1
  abc to dq0/1 -> Demux1/1
  Ground/1 -> Mux/3
  wL/1 -> Sum3/1
  PLL (3ph)/2 -> abc to dq0/2, abc to dq1/2, dq0 to abc/2
  Gain/1 -> Sum2/2
  dq0 to abc/1 -> Gain2/1
  Demux1/1 -> Sum4/2
  Sum1/1 -> Iq PI Controller/1
  Vgrid/1 -> Gain4/1
  Sum/1 -> Id PI Controller/1
  Demux1/3 -> Terminator2/1
  abc to dq1/1 -> Demux/1
  Sum2/1 -> Sum4/1
  Mux/1 -> dq0 to abc/1
  Demux1/2 -> Sum5/1
  Sum3/1 -> Sum5/2
  Gain3/1 -> Sum1/2
  Sum5/1 -> Mux/2
  Demux/1 -> wL/1, Sum/2
  Iq PI Controller/1 -> Sum3/2
  Sum4/1 -> Mux/1
  PLL (3ph)/1 -> Terminator/1
  Demux/2 -> Sum1/1, Gain/1
  Demux/3 -> Terminator1/1
  Iinv/1 -> Gain5/1
  Gain1/1 -> Sum/1
  Id/1 -> Gain7/1
  Iq/1 -> Gain6/1
  Gain4/1 -> abc to dq0/1, PLL (3ph)/1
  Gain5/1 -> abc to dq1/1
  Gain6/1 -> Gain3/1
  Gain7/1 -> Gain1/1
  Gain2/1 -> Uref/1

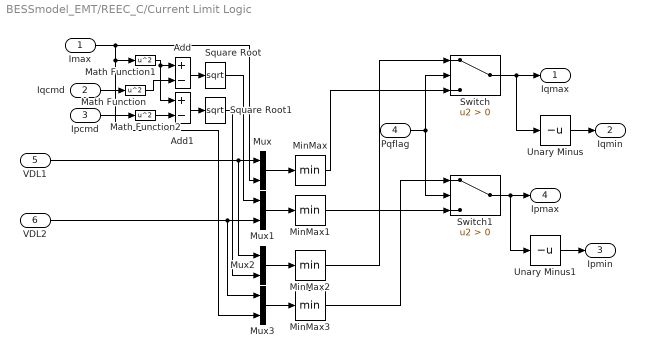
== system BESSmodel_EMT/REEC_C/Current Limit Logic ==
  Imax : Inport
  Iqcmd : Inport  Port=2
  Ipcmd : Inport  Port=3
  Pqflag : Inport  Port=4
  VDL1 : Inport  Port=5
  VDL2 : Inport  Port=6
  Add : Sum  Inputs=+-
  Add1 : Sum  Inputs=+-
  Math Function : Math  Operator=square  SaturateOnIntegerOverflow=on
  Math Function1 : Math  Operator=square  SaturateOnIntegerOverflow=on
  Math Function2 : Math  Operator=square  SaturateOnIntegerOverflow=on
  MinMax{,1..3} (4 alike) : MinMax
  Mux{,1..3} (4 alike) : Mux  Inputs=2
  Square Root : Sqrt  SaturateOnIntegerOverflow=on
  Square Root1 : Sqrt  SaturateOnIntegerOverflow=on
  Switch : Switch  Criteria=u2 > Threshold
  Switch1 : Switch  Criteria=u2 > Threshold
  Unary Minus : UnaryMinus
  Unary Minus1 : UnaryMinus
  Iqmax : Outport
  Iqmin : Outport  Port=2
  Ipmin : Outport  Port=3
  Ipmax : Outport  Port=4
  wires:
  MinMax3/1 -> Switch1/1
  MinMax1/1 -> Switch1/3
  VDL2/1 -> Mux3/1, Mux1/2
  Add/1 -> Square Root/1
  Imax/1 -> Mux3/2, Math Function1/1, Mux/2
  Pqflag/1 -> Switch/2, Switch1/2
  Square Root/1 -> Mux1/1
  MinMax2/1 -> Switch/1
  Add1/1 -> Square Root1/1
  Mux2/1 -> MinMax2/1
  Math Function2/1 -> Add1/2
  Mux3/1 -> MinMax3/1
  Ipcmd/1 -> Math Function2/1
  Square Root1/1 -> Mux2/2
  MinMax/1 -> Switch/3
  Math Function1/1 -> Add1/1, Add/1
  VDL1/1 -> Mux2/1, Mux/1
  Mux1/1 -> MinMax1/1
  Mux/1 -> MinMax/1
  Iqcmd/1 -> Math Function/1
  Math Function/1 -> Add/2
  Switch/1 -> Unary Minus/1, Iqmax/1
  Unary Minus/1 -> Iqmin/1
  Switch1/1 -> Unary Minus1/1, Ipmax/1
  Unary Minus1/1 -> Ipmin/1
